simulink model "anglesimu"  (R2015a)
settings: Solver=ode1  StartTime=0.0  StopTime=ts(end)  FixedStep=ts(2)-ts(1)  RelTol=1e-3
libraries: simulink x1, cstblocks x1
settings Model: Creator=roevhat  LastModifiedBy=roevhat
settings DataIOCC: ExternalInput=[ts, us]  LimitDataPoints=off  LoadExternalInput=on  OutputSaveName=ysimu

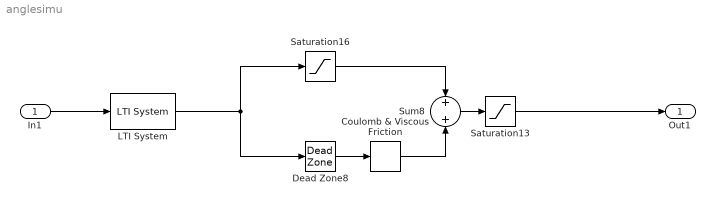
== system anglesimu ==
  In1 : Inport
  Coulomb & Viscous Friction : simulink/Discontinuities/Coulomb & Viscous Friction  offset=[0.165]  gain=1
  Dead Zone8 : DeadZone  LowerValue=-0.3225  UpperValue=0.337  SaturateOnIntegerOverflow=on
  LTI System : cstblocks/LTI System  sys=W  IC=[]
  Saturation13 : Saturate  UpperLimit=0.664  LowerLimit=-0.68
  Saturation16 : Saturate  UpperLimit=.326  LowerLimit=-0.224
  Sum8 : Sum  Inputs=+|+
  Out1 : Outport
  wires:
  In1/1 -> LTI System/1
  Dead Zone8/1 -> Coulomb & Viscous Friction/1
  Sum8/1 -> Saturation13/1
  Saturation16/1 -> Sum8/1
  Coulomb & Viscous Friction/1 -> Sum8/2
  LTI System/1 -> Dead Zone8/1, Saturation16/1
  Saturation13/1 -> Out1/1
